simulink model "DT_A_DIOL_BicopterSim"  (R2023a)
settings: Solver=ode4  StartTime=0.0  StopTime=Tend  FixedStep=Ts_sim  RelTol=1e-3
values from neighbouring files (symbols this model uses):
  alpha_1 = 0.2    [A_DIOL_sim_runner.m]    (also in DT_A_DIOL_sim_runner.m)
  alpha_2 = 1.2    [A_DIOL_sim_runner.m]    (also in DT_A_DIOL_sim_runner.m)
  c_1 = 6    [A_DIOL_sim_runner.m]    (also in DT_A_DIOL_sim_runner.m)
  c_2 = 3    [A_DIOL_sim_runner.m]    (also in DT_A_DIOL_sim_runner.m)
  g = 9.81    [A_DIOL_sim_runner.m]    (also in DT_A_DIOL_sim_runner.m)
  gamma = 10    [A_DIOL_sim_runner.m]    (also in DT_A_DIOL_sim_runner.m)
  J = 0.05    [A_DIOL_sim_runner.m]    (also in DT_A_DIOL_sim_runner.m)
  J_hat_0 = 0.1    [A_DIOL_sim_runner.m]    (also in DT_A_DIOL_sim_runner.m)
  kd = place(Ad,Bd,pd)    [DT_A_DIOL_sim_runner.m]
  lambda = 80    [A_DIOL_sim_runner.m]    (also in DT_A_DIOL_sim_runner.m = 40)
  m = 1    [A_DIOL_sim_runner.m]    (also in DT_A_DIOL_sim_runner.m)
  m_hat_0 = 0.5    [A_DIOL_sim_runner.m]    (also in DT_A_DIOL_sim_runner.m)
  Phibar_0 = ones(2,2)    [A_DIOL_sim_runner.m]    (also in DT_A_DIOL_sim_runner.m)
  Phif_0 = zeros(6,2)    [A_DIOL_sim_runner.m]    (also in DT_A_DIOL_sim_runner.m)
  Psi_int_0 = [0;0;0;0;0;0]    [A_DIOL_sim_runner.m]    (also in DT_A_DIOL_sim_runner.m)
  r1_ref_0 = (r1_ref(1,2:6))'    [DT_A_DIOL_sim_runner.m]
  r2_ref_0 = (r2_ref(1,2:6))'    [DT_A_DIOL_sim_runner.m]
  Theta_hat_0 = [1/m_hat_0; 1/J_hat_0]    [A_DIOL_sim_runner.m]    (also in DT_A_DIOL_sim_runner.m)
  Ts = 1e-4    (= 0.0001)    [A_DIOL_sim_runner.m]    (also in DT_A_DIOL_sim_runner.m = 0.01; trajectory_csv_generator.m)
  u1_0 = g*m_hat_0    (= 4.905)    [A_DIOL_sim_runner.m]    (also in DT_A_DIOL_sim_runner.m)
  u1_dot_0 = 0    [A_DIOL_sim_runner.m]    (also in DT_A_DIOL_sim_runner.m)
  u_0 = [u1_0; 0]    [DT_A_DIOL_sim_runner.m]
  x0 = [0.01; 0.00; 0.03; 0.02; 0.01; 0.00]    [A_DIOL_sim_runner.m]    (also in DT_A_DIOL_sim_runner.m)
  Xbar_0 = zeros(2,1)    [A_DIOL_sim_runner.m]    (also in DT_A_DIOL_sim_runner.m)
  xf_0 = x0    [A_DIOL_sim_runner.m]    (also in DT_A_DIOL_sim_runner.m)
undefined symbols (not defined in the file or in its folder): DiscIntNeverNeededParam
settings Model: Creator=PhDstudent1  LastModifiedBy=Juan Augusto Paredes
settings ModelReferenceCC: EnableRefExpFcnMdlSchedulingChecks=on

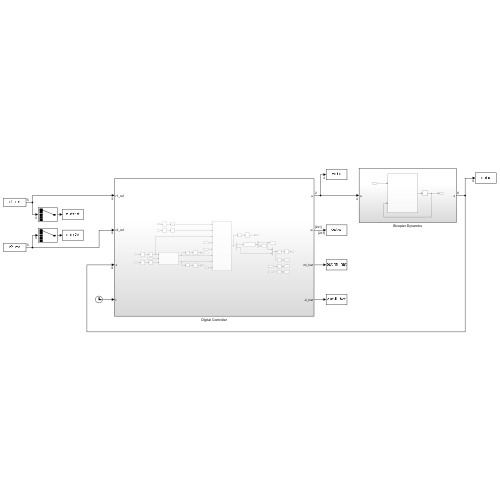
[thumbnail: Simulink's stored preview of the top-level diagram]
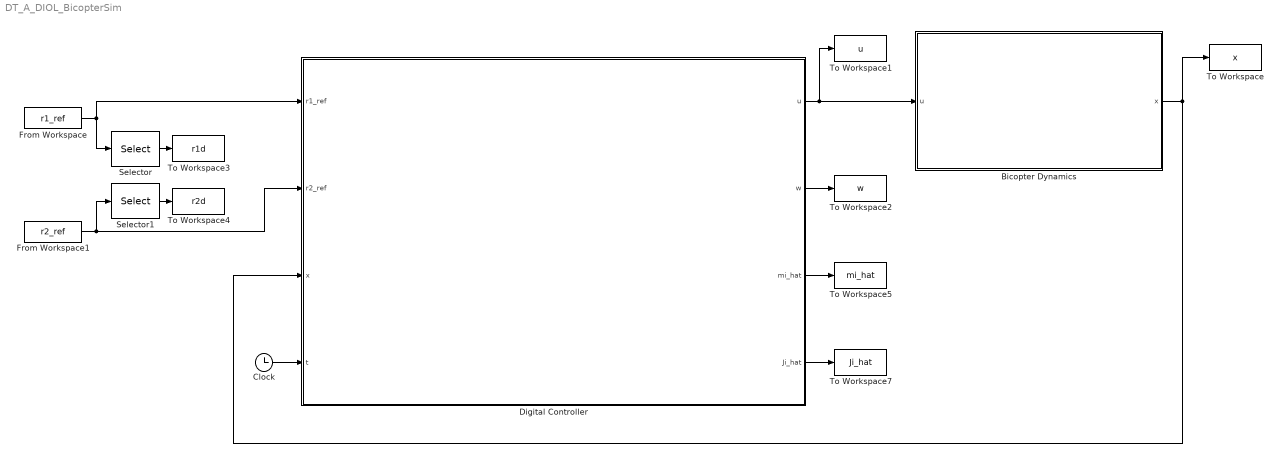
== system DT_A_DIOL_BicopterSim ==
  Bicopter Dynamics : Subsystem
  Clock : Clock
  Digital Controller : Subsystem
  From Workspace : FromWorkspace  VariableName=r1_ref  SampleTime=Ts
  From Workspace1 : FromWorkspace  VariableName=r2_ref  SampleTime=Ts
  Selector : Selector  InputPortWidth=5  IndexOptions=Index vector (dialog)  Indices=[1]  OutputSizes=1
  Selector1 : Selector  InputPortWidth=5  IndexOptions=Index vector (dialog)  Indices=[1]  OutputSizes=1
  To Workspace : ToWorkspace  VariableName=x  SampleTime=-1
  To Workspace1 : ToWorkspace  VariableName=u  SampleTime=-1
  To Workspace2 : ToWorkspace  VariableName=w  SampleTime=-1
  To Workspace3 : ToWorkspace  VariableName=r1d  SampleTime=-1
  To Workspace4 : ToWorkspace  VariableName=r2d  SampleTime=-1
  To Workspace5 : ToWorkspace  VariableName=mi_hat  SampleTime=-1
  To Workspace7 : ToWorkspace  VariableName=Ji_hat  SampleTime=-1
  wires:
  Bicopter Dynamics/1(x) -> To Workspace/1, Digital Controller/3(x)
  From Workspace/1 -> Selector/1, Digital Controller/1(r1_ref)
  From Workspace1/1 -> Digital Controller/2(r2_ref), Selector1/1
  Selector/1 -> To Workspace3/1
  Selector1/1 -> To Workspace4/1
  Digital Controller/4(Ji_hat) -> To Workspace7/1
  Digital Controller/3(mi_hat) -> To Workspace5/1
  Digital Controller/2(w) -> To Workspace2/1
  Digital Controller/1(u) -> Bicopter Dynamics/1(u), To Workspace1/1
  Clock/1 -> Digital Controller/4(t)

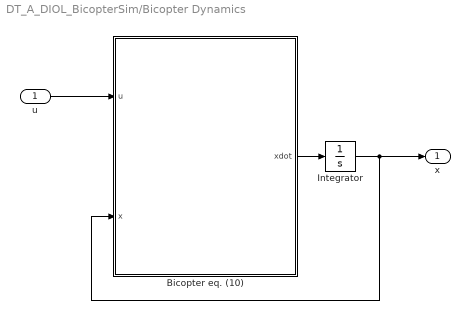
== system DT_A_DIOL_BicopterSim/Bicopter Dynamics ==
  u : Inport
  Bicopter eq. (10) : MATLAB Function  TreatAsAtomicUnit=on
  Integrator : Integrator  InitialCondition=x0
  x : Outport
  wires:
  Bicopter eq. (10)/1(xdot) -> Integrator/1
  u/1 -> Bicopter eq. (10)/1(u)
  Integrator/1 -> x/1, Bicopter eq. (10)/2(x)

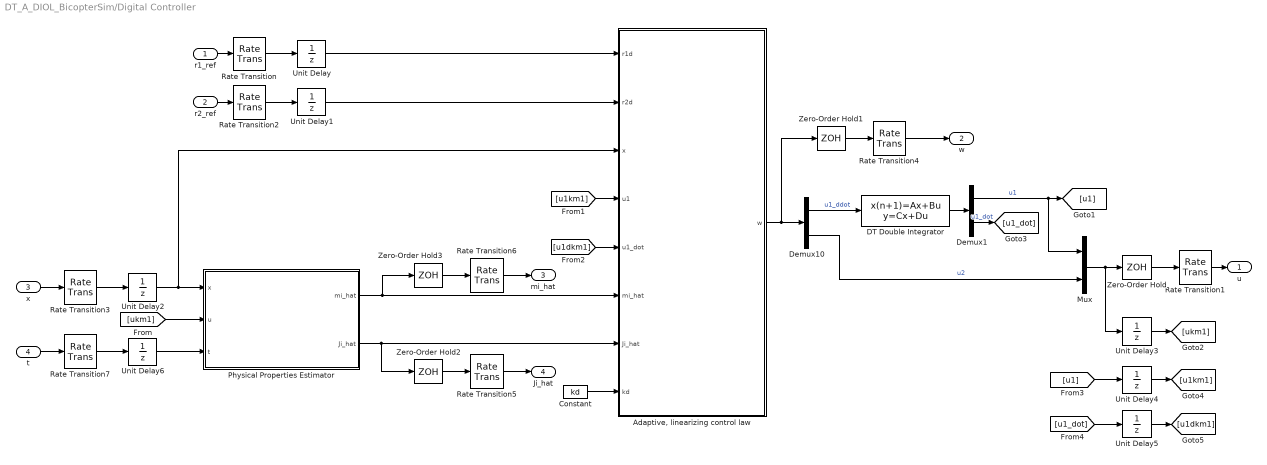
== system DT_A_DIOL_BicopterSim/Digital Controller ==
  r1_ref : Inport
  r2_ref : Inport  Port=2
  x : Inport  Port=3
  t : Inport  Port=4
  "Adaptive, linearizing control law" : Subsystem
  Constant : Constant  Value=kd
  DT Double Integrator : DiscreteStateSpace  A=[1 Ts; 0 1]  B=[0.5*(Ts^2); Ts]  C=eye(2)  D=[0; 0]  InitialCondition=[u1_0; u1_dot_0]  SampleTime=Ts
  Demux1 : Demux  Outputs=2
  Demux10 : Demux  Outputs=2
  Mux : Mux  Inputs=2
  Physical Properties Estimator : Subsystem
  Rate Transition : RateTransition  InitialCondition=r1_ref_0
  Rate Transition1 : RateTransition  InitialCondition=u_0
  Rate Transition2 : RateTransition  InitialCondition=r2_ref_0
  Rate Transition3 : RateTransition  InitialCondition=x0
  Rate Transition4 : RateTransition  InitialCondition=[0;0]
  Rate Transition5 : RateTransition  InitialCondition=1/J_hat_0
  Rate Transition6 : RateTransition  InitialCondition=1/m_hat_0
  Rate Transition7 : RateTransition
  Unit Delay : UnitDelay  InitialCondition=r1_ref_0  SampleTime=Ts  HasFrameUpgradeWarning=on
  Unit Delay1 : UnitDelay  InitialCondition=r2_ref_0  SampleTime=Ts  HasFrameUpgradeWarning=on
  Unit Delay2 : UnitDelay  InitialCondition=x0  SampleTime=Ts  HasFrameUpgradeWarning=on
  Unit Delay3 : UnitDelay  InitialCondition=u_0  SampleTime=Ts  HasFrameUpgradeWarning=on
  Unit Delay4 : UnitDelay  InitialCondition=u1_0  SampleTime=Ts  HasFrameUpgradeWarning=on
  Unit Delay5 : UnitDelay  InitialCondition=u1_dot_0  SampleTime=Ts  HasFrameUpgradeWarning=on
  Unit Delay6 : UnitDelay  SampleTime=Ts  HasFrameUpgradeWarning=on
  Zero-Order Hold{,1..3} (4 alike) : ZeroOrderHold  SampleTime=Ts
  u : Outport
  w : Outport  Port=2
  mi_hat : Outport  Port=3
  Ji_hat : Outport  Port=4
  wires:
  Rate Transition/1 -> Unit Delay/1
  Rate Transition2/1 -> Unit Delay1/1
  x/1 -> Rate Transition3/1
  Rate Transition3/1 -> Unit Delay2/1
  Zero-Order Hold/1 -> Rate Transition1/1
  r1_ref/1 -> Rate Transition/1
  Rate Transition1/1 -> u/1
  r2_ref/1 -> Rate Transition2/1
  Unit Delay3/1 -> [ukm1]
  Unit Delay2/1 -> "Adaptive, linearizing control law"/3(x), Physical Properties Estimator/1(x)
  [ukm1] -> Physical Properties Estimator/2(u)
  Unit Delay/1 -> "Adaptive, linearizing control law"/1(r1d)
  Unit Delay1/1 -> "Adaptive, linearizing control law"/2(r2d)
  [u1km1] -> "Adaptive, linearizing control law"/4(u1)
  [u1dkm1] -> "Adaptive, linearizing control law"/5(u1_dot)
  Physical Properties Estimator/1(mi_hat) -> Zero-Order Hold3/1, "Adaptive, linearizing control law"/6(mi_hat)
  Physical Properties Estimator/2(Ji_hat) -> Zero-Order Hold2/1, "Adaptive, linearizing control law"/7(Ji_hat)
  Constant/1 -> "Adaptive, linearizing control law"/8(kd)
  Demux10/1 -> DT Double Integrator/1  "u1_ddot"
  DT Double Integrator/1 -> Demux1/1
  Mux/1 -> Unit Delay3/1, Zero-Order Hold/1
  Demux10/2 -> Mux/2  "u2"
  Demux1/1 -> [u1], Mux/1  "u1"
  Demux1/2 -> [u1_dot]  "u1_dot"
  [u1] -> Unit Delay4/1
  [u1_dot] -> Unit Delay5/1
  Unit Delay4/1 -> [u1km1]
  Unit Delay5/1 -> [u1dkm1]
  Zero-Order Hold1/1 -> Rate Transition4/1
  Rate Transition4/1 -> w/1
  "Adaptive, linearizing control law"/1(w) -> Zero-Order Hold1/1, Demux10/1
  Zero-Order Hold2/1 -> Rate Transition5/1
  Zero-Order Hold3/1 -> Rate Transition6/1
  Rate Transition6/1 -> mi_hat/1
  Rate Transition5/1 -> Ji_hat/1
  t/1 -> Rate Transition7/1
  Rate Transition7/1 -> Unit Delay6/1
  Unit Delay6/1 -> Physical Properties Estimator/3(t)

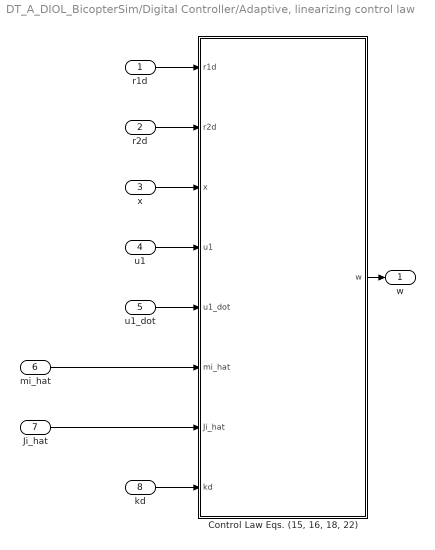
== system DT_A_DIOL_BicopterSim/Digital Controller/Adaptive, linearizing control law ==
  r1d : Inport
  r2d : Inport  Port=2
  x : Inport  Port=3
  u1 : Inport  Port=4
  u1_dot : Inport  Port=5
  mi_hat : Inport  Port=6
  Ji_hat : Inport  Port=7
  kd : Inport  Port=8
  "Control Law Eqs. (15, 16, 18, 22)" : MATLAB Function  TreatAsAtomicUnit=on
  w : Outport
  wires:
  r2d/1 -> "Control Law Eqs. (15, 16, 18, 22)"/2(r2d)
  x/1 -> "Control Law Eqs. (15, 16, 18, 22)"/3(x)
  "Control Law Eqs. (15, 16, 18, 22)"/1(w) -> w/1
  u1_dot/1 -> "Control Law Eqs. (15, 16, 18, 22)"/5(u1_dot)
  kd/1 -> "Control Law Eqs. (15, 16, 18, 22)"/8(kd)
  u1/1 -> "Control Law Eqs. (15, 16, 18, 22)"/4(u1)
  r1d/1 -> "Control Law Eqs. (15, 16, 18, 22)"/1(r1d)
  mi_hat/1 -> "Control Law Eqs. (15, 16, 18, 22)"/6(mi_hat)
  Ji_hat/1 -> "Control Law Eqs. (15, 16, 18, 22)"/7(Ji_hat)

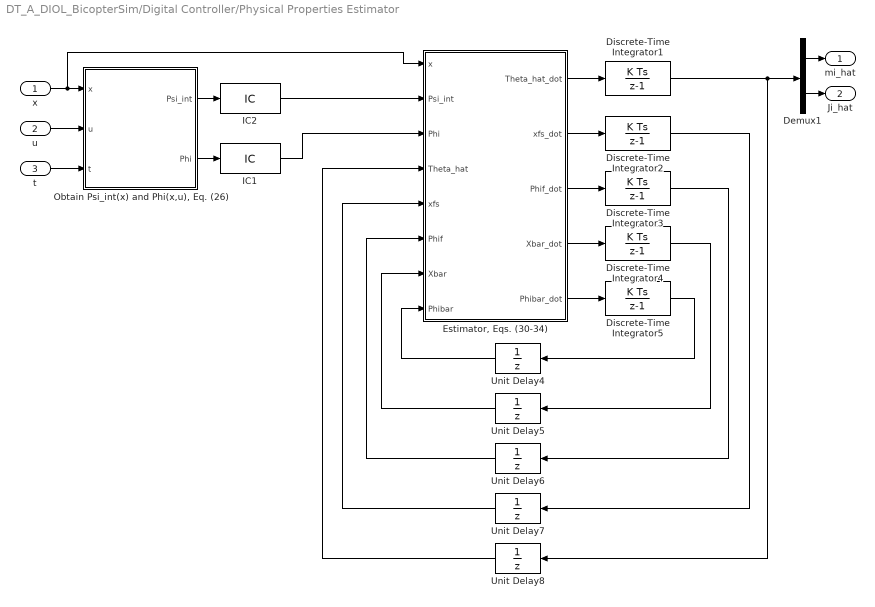
== system DT_A_DIOL_BicopterSim/Digital Controller/Physical Properties Estimator ==
  x : Inport
  u : Inport  Port=2
  t : Inport  Port=3
  Demux1 : Demux  Outputs=2
  Discrete-Time Integrator1 : DiscreteIntegrator  InitialCondition=Theta_hat_0  SampleTime=Ts  ICPrevOutput=DiscIntNeverNeededParam  ICPrevScaledInput=DiscIntNeverNeededParam
  Discrete-Time Integrator2 : DiscreteIntegrator  InitialCondition=xf_0 - x0 + Psi_int_0  SampleTime=Ts  ICPrevOutput=DiscIntNeverNeededParam  ICPrevScaledInput=DiscIntNeverNeededParam
  Discrete-Time Integrator3 : DiscreteIntegrator  InitialCondition=Phif_0  SampleTime=Ts  ICPrevOutput=DiscIntNeverNeededParam  ICPrevScaledInput=DiscIntNeverNeededParam
  Discrete-Time Integrator4 : DiscreteIntegrator  InitialCondition=Xbar_0  SampleTime=Ts  ICPrevOutput=DiscIntNeverNeededParam  ICPrevScaledInput=DiscIntNeverNeededParam
  Discrete-Time Integrator5 : DiscreteIntegrator  InitialCondition=Phibar_0  SampleTime=Ts  ICPrevOutput=DiscIntNeverNeededParam  ICPrevScaledInput=DiscIntNeverNeededParam
  "Estimator, Eqs. (30-34)" : MATLAB Function  TreatAsAtomicUnit=on
  IC1 : InitialCondition  Value=zeros(6,2)
  IC2 : InitialCondition  Value=Psi_int_0
  "Obtain Psi_int(x) and Phi(x,u), Eq. (26)" : MATLAB Function  TreatAsAtomicUnit=on
  Unit Delay4 : UnitDelay  InitialCondition=Phibar_0  SampleTime=Ts  HasFrameUpgradeWarning=on
  Unit Delay5 : UnitDelay  InitialCondition=Xbar_0  SampleTime=Ts  HasFrameUpgradeWarning=on
  Unit Delay6 : UnitDelay  InitialCondition=Phif_0  SampleTime=Ts  HasFrameUpgradeWarning=on
  Unit Delay7 : UnitDelay  InitialCondition=xf_0 - x0 + Psi_int_0  SampleTime=Ts  HasFrameUpgradeWarning=on
  Unit Delay8 : UnitDelay  InitialCondition=Theta_hat_0  SampleTime=Ts  HasFrameUpgradeWarning=on
  mi_hat : Outport
  Ji_hat : Outport  Port=2
  wires:
  Unit Delay5/1 -> "Estimator, Eqs. (30-34)"/7(Xbar)
  "Estimator, Eqs. (30-34)"/2(xfs_dot) -> Discrete-Time Integrator2/1
  x/1 -> "Estimator, Eqs. (30-34)"/1(x), "Obtain Psi_int(x) and Phi(x,u), Eq. (26)"/1(x)
  Unit Delay7/1 -> "Estimator, Eqs. (30-34)"/5(xfs)
  Discrete-Time Integrator1/1 -> Demux1/1, Unit Delay8/1
  Discrete-Time Integrator4/1 -> Unit Delay5/1
  "Estimator, Eqs. (30-34)"/4(Xbar_dot) -> Discrete-Time Integrator4/1
  "Estimator, Eqs. (30-34)"/1(Theta_hat_dot) -> Discrete-Time Integrator1/1
  "Obtain Psi_int(x) and Phi(x,u), Eq. (26)"/1(Psi_int) -> IC2/1
  Unit Delay4/1 -> "Estimator, Eqs. (30-34)"/8(Phibar)
  Unit Delay6/1 -> "Estimator, Eqs. (30-34)"/6(Phif)
  Unit Delay8/1 -> "Estimator, Eqs. (30-34)"/4(Theta_hat)
  Discrete-Time Integrator2/1 -> Unit Delay7/1
  "Estimator, Eqs. (30-34)"/3(Phif_dot) -> Discrete-Time Integrator3/1
  IC1/1 -> "Estimator, Eqs. (30-34)"/3(Phi)
  Discrete-Time Integrator3/1 -> Unit Delay6/1
  Discrete-Time Integrator5/1 -> Unit Delay4/1
  "Obtain Psi_int(x) and Phi(x,u), Eq. (26)"/2(Phi) -> IC1/1
  Demux1/2 -> Ji_hat/1
  "Estimator, Eqs. (30-34)"/5(Phibar_dot) -> Discrete-Time Integrator5/1
  Demux1/1 -> mi_hat/1
  u/1 -> "Obtain Psi_int(x) and Phi(x,u), Eq. (26)"/2(u)
  IC2/1 -> "Estimator, Eqs. (30-34)"/2(Psi_int)
  t/1 -> "Obtain Psi_int(x) and Phi(x,u), Eq. (26)"/3(t)

== matlab function DT_A_DIOL_BicopterSim/Digital Controller/Physical Properties Estimator/Obtain Psi_int(x) and Phi(x,u), Eq. (26) ==
  settings: updateMethod=DISCRETE  sampleTime=Ts
  data: x input size=6; u input size=2; t input size=1; Psi_int output size=6; Phi output size=[6,2]; g parameter size=1
function [Psi_int, Phi] = x_2_Psi_Phi(x,u,t,g)
    Psi_int = [x(1);...
          x(2);...
          x(3);...
          0;...
          -g*t;...
          0];
    Phi = [0 0;...
          0 0;...
          0 0;...
          -u(1)*sin(x(3)) 0;...
          u(1)*cos(x(3)) 0;...
          0 u(2)];
end

== matlab function DT_A_DIOL_BicopterSim/Digital Controller/Physical Properties Estimator/Estimator, Eqs. (30-34) ==
  settings: updateMethod=DISCRETE  sampleTime=Ts
  data: Theta_hat_dot output size=2; xfs_dot output size=6; Phif_dot output size=[6,2]; x input size=6; Psi_int input size=6; Phi input size=[6, 2]; Theta_hat input size=2; xfs input size=6; Phif input size=[6,2]; Xbar input size=2; Phibar input size=[2 2]; Xbar_dot output size=2; Phibar_dot output size=[2 2]; gamma parameter size=1; lambda parameter size=1; c_1 parameter size=1; c_2 parameter size=1; alpha_1 parameter size=1; alpha_2 parameter size=1
function [Theta_hat_dot,xfs_dot,Phif_dot,...
    Xbar_dot,Phibar_dot] = estimator(x, Psi_int,Phi,...
                                        Theta_hat,xfs,Phif,Xbar,Phibar,...
                                        gamma, lambda, c_1, c_2, alpha_1, alpha_2)

%xf and Phif dynamics, Eq. (30)

xf = xfs + x - Psi_int; % xfs is an intermediate variable for calculating xf
xfs_dot=-gamma*xf;

Phif_dot=-gamma*Phif+Phi;

%Finite time estimator

Xbar_dot = Phif'*xf - lambda*Xbar; % Eq. (33)
Phibar_dot = Phif'*Phif - lambda*Phibar; % Eq. (34)
grad= Phibar*Theta_hat-Xbar; % Eq. (32)
Theta_hat_dot = -c_1*grad/(norm(grad)^(1-alpha_1))-c_2*grad/(norm(grad)^(1-alpha_2));  % Eq. (31)

end

== matlab function DT_A_DIOL_BicopterSim/Digital Controller/Adaptive, linearizing control law/Control Law Eqs. (15, 16, 18, 22) ==
  settings: updateMethod=DISCRETE  sampleTime=Ts
  data: r1d input; r2d input; x input size=6; u1 input size=1; u1_dot input size=1; w output; mi_hat input; Ji_hat input; kd input; g parameter size=1
function w = control_law(r1d, r2d, x, u1, u1_dot, mi_hat, Ji_hat, kd, g)

m_hat = 1/mi_hat;
J_hat = 1/Ji_hat;

% Assembling \chi vector, Eq. (11)
Chi = [x;u1;u1_dot];

% Assembling \Xi vector, Eq. (20)
E = [Chi(1);...
    Chi(4);...
    -sin(Chi(3))*Chi(7)/m_hat;...
    -cos(Chi(3))*Chi(6)*Chi(7)/m_hat - sin(Chi(3))*Chi(8)/m_hat;...
    Chi(2);...
    Chi(5);...
    -g + cos(Chi(3))*Chi(7)/m_hat;...
    -sin(Chi(3))*Chi(6)*Chi(7)/m_hat + cos(Chi(3))*Chi(8)/m_hat];

Ed = [r1d(1:4); r2d(1:4)];
v = kd*(E - Ed) + [r1d(5); r2d(5)]; % Eq. (22)

alpha_X =[-2*Chi(8)*cos(Chi(3))+Chi(6)*Chi(7)*sin(Chi(3)); -2*Chi(8)*sin(Chi(3))-Chi(6)*Chi(7)*cos(Chi(3))].*Chi(6)./m_hat ; % Eq. (16)
beta_X_inv = [-m_hat*sin(Chi(3)), m_hat*cos(Chi(3)); -J_hat*m_hat*cos(Chi(3))/Chi(7), -J_hat*m_hat*sin(Chi(3))/Chi(7)]; % Eq. (18)

w = beta_X_inv*(alpha_X-v); % Eq. (15)

end

== matlab function DT_A_DIOL_BicopterSim/Bicopter Dynamics/Bicopter eq. (10) ==
  data: u input size=2; xdot output size=6; x input size=6; m parameter size=1; g parameter size=1; J parameter size=1
function xdot  = bicopter_dyn(u,x,m, g, J)

xdot = [x(4);...
        x(5);...
        x(6);...
        -sin(x(3))*u(1)/m;...
        -g+cos(x(3))*u(1)/m;...
        u(2)/J];

end
